simulink model "Enable_Lab3_System_Modeling"  (R2024b)
settings: Solver=FixedStepDiscrete  StartTime=0.0  StopTime=10.0  FixedStep=1e-3  RelTol=1e-3
libraries: simulink x1, dspswit3 x1
settings Model: Creator=Ahmad  LastModifiedBy=Ahmad
settings DebuggingCC: AlgebraicLoopMsg=none

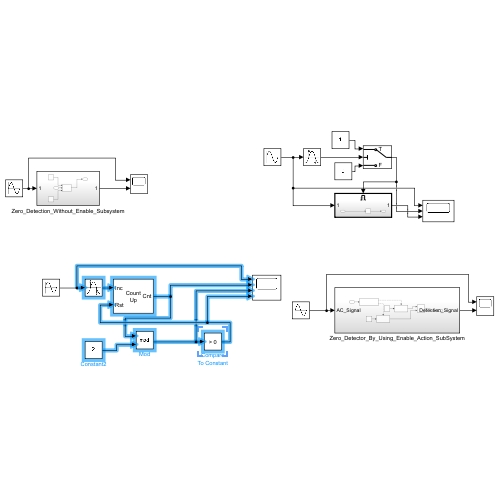
[thumbnail: Simulink's stored preview of the top-level diagram]
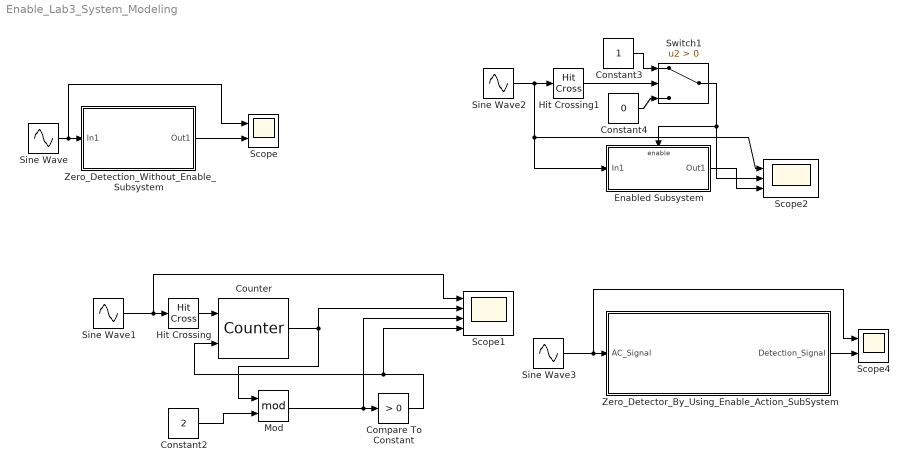
== system Enable_Lab3_System_Modeling ==
  Compare To Constant : simulink/Logic and Bit Operations/Compare To Constant  relop=>  const=0  OutDataTypeStr=boolean
  Constant2 : Constant  Value=2
  Constant3 : Constant
  Constant4 : Constant  Value=0
  Counter : dspswit3/Counter  Direction=Up  CountEvent=Rising edge  CounterSize=User defined  MaxCount=255  InitialCount=0  Output=Count  HitValue=32  ResetInput=on  SamplesPerFrame=1  Ts=1  CntDtype=double  HitDtype=Logical
  Enabled Subsystem : Subsystem  TreatAsAtomicUnit=on
  Hit Crossing : HitCross
  Hit Crossing1 : HitCross
  Mod : Math  Operator=mod
  Scope : Scope  NumInputPorts=2
  Scope1 : Scope  NumInputPorts=4
  Scope2 : Scope  NumInputPorts=3
  Scope4 : Scope  NumInputPorts=2
  Sine Wave : Sin  SampleTime=0
  Sine Wave1 : Sin  SampleTime=0
  Sine Wave2 : Sin  Frequency=2*pi*0.5  SampleTime=0
  Sine Wave3 : Sin  Frequency=2*pi*0.5  SampleTime=0
  Switch1 : Switch  Criteria=u2 > Threshold  SaturateOnIntegerOverflow=off  InputSameDT=off
  Zero_Detection_Without_Enable_Subsystem : Subsystem
  Zero_Detector_By_Using_Enable_Action_SubSystem : Subsystem
  wires:
  Sine Wave/1 -> Scope/1, Zero_Detection_Without_Enable_Subsystem/1(In1)
  Sine Wave1/1 -> Scope1/1, Hit Crossing/1
  Hit Crossing/1 -> Counter/1
  Counter/1 -> Mod/1, Scope1/2
  Compare To Constant/1 -> Scope1/4, Counter/2
  Sine Wave2/1 -> Enabled Subsystem/1(In1), Scope2/1, Hit Crossing1/1
  Enabled Subsystem/1(Out1) -> Scope2/3
  Hit Crossing1/1 -> Switch1/2
  Constant3/1 -> Switch1/1
  Constant4/1 -> Switch1/3
  Switch1/1 -> Scope2/2, Enabled Subsystem/Enable
  Mod/1 -> Scope1/3, Compare To Constant/1
  Sine Wave3/1 -> Scope4/1, Zero_Detector_By_Using_Enable_Action_SubSystem/1(AC_Signal)
  Zero_Detector_By_Using_Enable_Action_SubSystem/1(Detection_Signal) -> Scope4/2
  Constant2/1 -> Mod/2
  Zero_Detection_Without_Enable_Subsystem/1(Out1) -> Scope/2

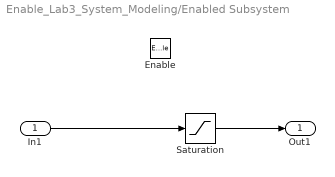
== system Enable_Lab3_System_Modeling/Enabled Subsystem ==
  In1 : Inport
  Enable : EnablePort
  Saturation : Saturate  UpperLimit=1  LowerLimit=0
  Out1 : Outport
  wires:
  In1/1 -> Saturation/1
  Saturation/1 -> Out1/1

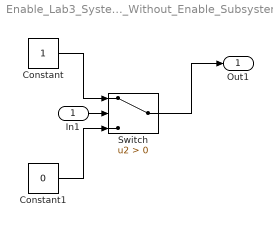
== system Enable_Lab3_System_Modeling/Zero_Detection_Without_Enable_Subsystem ==
  In1 : Inport
  Constant : Constant
  Constant1 : Constant  Value=0
  Switch : Switch  Criteria=u2 > Threshold  SaturateOnIntegerOverflow=off  InputSameDT=off
  Out1 : Outport
  wires:
  Constant/1 -> Switch/1
  Constant1/1 -> Switch/3
  In1/1 -> Switch/2
  Switch/1 -> Out1/1

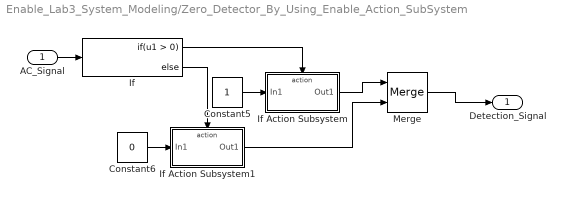
== system Enable_Lab3_System_Modeling/Zero_Detector_By_Using_Enable_Action_SubSystem ==
  AC_Signal : Inport
  Constant5 : Constant
  Constant6 : Constant  Value=0
  If : If
  If Action Subsystem : Subsystem  TreatAsAtomicUnit=on
  If Action Subsystem1 : Subsystem  TreatAsAtomicUnit=on
  Merge : Merge
  Detection_Signal : Outport
  wires:
  Constant5/1 -> If Action Subsystem/1(In1)
  Constant6/1 -> If Action Subsystem1/1(In1)
  If Action Subsystem/1(Out1) -> Merge/1
  If/2 -> If Action Subsystem1/Action
  Merge/1 -> Detection_Signal/1
  If/1 -> If Action Subsystem/Action
  AC_Signal/1 -> If/1
  If Action Subsystem1/1(Out1) -> Merge/2

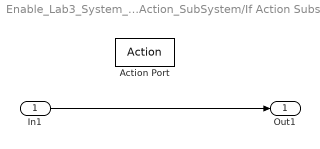
== system Enable_Lab3_System_Modeling/Zero_Detector_By_Using_Enable_Action_SubSystem/If Action Subsystem ==
  In1 : Inport
  Action Port : ActionPort  ActionPortLabel=if(u1 > 0)
  Out1 : Outport
  wires:
  In1/1 -> Out1/1

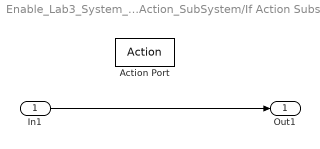
== system Enable_Lab3_System_Modeling/Zero_Detector_By_Using_Enable_Action_SubSystem/If Action Subsystem1 ==
  In1 : Inport
  Action Port : ActionPort  ActionPortLabel=else
  Out1 : Outport
  wires:
  In1/1 -> Out1/1
